simulink model "DC_Motor_Mathematical_Modelling"  (R2025a)
settings: Solver=ode23tb  StartTime=0.0  StopTime=10.0  MaxStep=1e-4  RelTol=1e-3
settings Model: Creator=Jawad  LastModifiedBy=Jawad

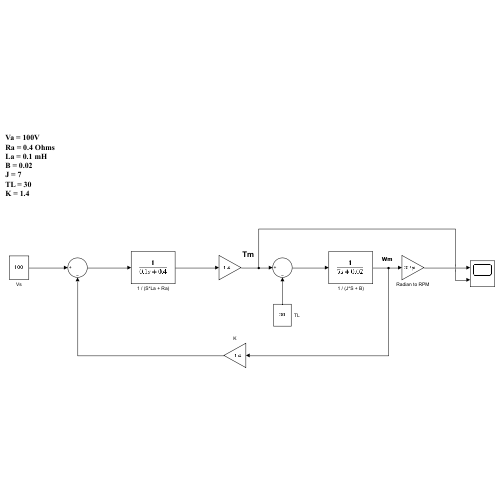
[thumbnail: Simulink's stored preview of the top-level diagram]
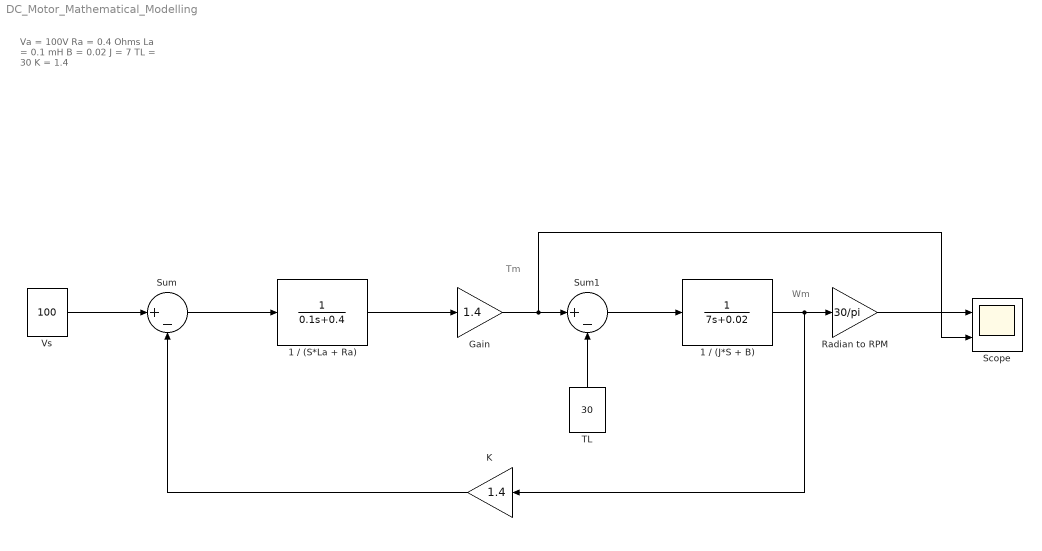
== system DC_Motor_Mathematical_Modelling ==
  note: Wm
  note: Tm
  note: Va = 100V
      | Ra = 0.4 Ohms
      | La = 0.1 mH
      | B = 0.02
      | J = 7
      | TL = 30
      | K = 1.4
  1 / (J*S + B) : TransferFcn  Denominator=[7 0.02]
  1 / (S*La + Ra) : TransferFcn  Denominator=[0.1 0.4]
  Gain : Gain  Gain=1.4
  K : Gain  Gain=1.4
  Radian to RPM : Gain  Gain=30/pi
  Scope : Scope  NumInputPorts=2
      settings: ActiveDisplayYMinimum=-78.131677568453568  ActiveDisplayYMaximum=698.67103530379211
  Sum : Sum  Inputs=|+-
  Sum1 : Sum  Inputs=|+-
  TL : Constant  Value=30
  Vs : Constant  Value=100
  wires:
  Sum/1 -> 1 / (S*La + Ra)/1
  1 / (S*La + Ra)/1 -> Gain/1
  Gain/1 -> Scope/2, Sum1/1
  Sum1/1 -> 1 / (J*S + B)/1
  1 / (J*S + B)/1 -> K/1, Radian to RPM/1
  Radian to RPM/1 -> Scope/1
  K/1 -> Sum/2
  Vs/1 -> Sum/1
  TL/1 -> Sum1/2
